simulink model "pro_newton1"  (R2022a)
settings: Solver=ode45  StartTime=0.0  StopTime=10.0  RelTol=1e-3
settings Model: Creator=55062  LastModifiedBy=55062
settings SolverCC: InitialStep=0.001

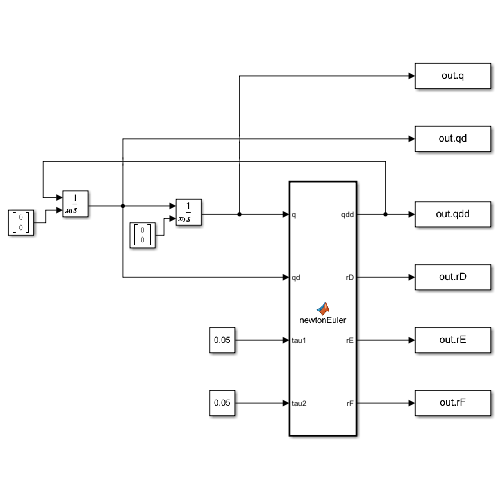
[thumbnail: Simulink's stored preview of the top-level diagram]
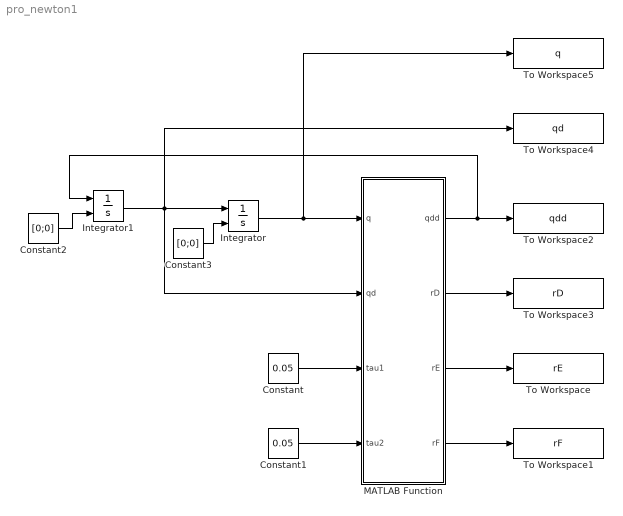
== system pro_newton1 ==
  Constant : Constant  Value=0.05
  Constant1 : Constant  Value=0.05
  Constant2 : Constant  Value=[0;0]  VectorParams1D=off
  Constant3 : Constant  Value=[0;0]  VectorParams1D=off
  Integrator : Integrator  InitialConditionSource=external
  Integrator1 : Integrator  InitialConditionSource=external
  MATLAB Function : MATLAB Function  TreatAsAtomicUnit=on
  To Workspace : ToWorkspace  VariableName=rE  SaveFormat=Timeseries  SampleTime=-1
  To Workspace1 : ToWorkspace  VariableName=rF  SaveFormat=Timeseries  SampleTime=-1
  To Workspace2 : ToWorkspace  VariableName=qdd  SaveFormat=Timeseries  SampleTime=-1
  To Workspace3 : ToWorkspace  VariableName=rD  SaveFormat=Timeseries  SampleTime=-1
  To Workspace4 : ToWorkspace  VariableName=qd  SaveFormat=Timeseries  SampleTime=-1
  To Workspace5 : ToWorkspace  VariableName=q  SaveFormat=Timeseries  SampleTime=-1
  wires:
  Integrator/1 -> To Workspace5/1, MATLAB Function/1(q)
  Integrator1/1 -> MATLAB Function/2(qd), To Workspace4/1, Integrator/1
  MATLAB Function/1(qdd) -> To Workspace2/1, Integrator1/1
  Constant/1 -> MATLAB Function/3(tau1)
  Constant1/1 -> MATLAB Function/4(tau2)
  MATLAB Function/3(rE) -> To Workspace/1
  MATLAB Function/4(rF) -> To Workspace1/1
  MATLAB Function/2(rD) -> To Workspace3/1
  Constant2/1 -> Integrator1/2
  Constant3/1 -> Integrator/2

== matlab function pro_newton1/MATLAB Function ==
  data: qdd output; rD output; q input; qd input; tau1 input; tau2 input; rE output; rF output
function [qdd,rD,rE,rF]  = newtonEuler(q,qd,tau1,tau2)
L0 = 0.5;
L1 = 0.15;
L2 = 0.1;
m1 = 0.6;
m2 = 0.5;
J1 = m1*L1^2/12;
J2 = m2*L2^2/12;
g = 9.8;
II = [0,-1;1,0];
ex = [1;0];

l1 = 0.05;
l2 = 0.025;

R1 = [cos(q(1)), -sin(q(1)); sin(q(1)), cos(q(1))];
R2 = [cos(q(2)), -sin(q(2)); sin(q(2)), cos(q(2))];
rC = [L0;0];
rD = rC - l1*R1*ex;
rE = rC + (L1 - l1)*R1*ex;
rF = rC - l1*R1*ex + L2*R2*ex/2;

J = [(L1/2-l1)*II*R1*ex, zeros(2,1);...
     1,                  0;...
     -l1*II*R1*ex,       (L2/2-l2)*II*R2*ex;...
     0,                  1];

C = [-(L1/2-l1)*R1*ex*(qd(1)^2);...
     0;...
     l1*R1*ex*(qd(1)^2) - (L2/2-l2)*R2*ex*(qd(2)^2);...
     0];

Phi = diag([m1,m1,J1,m2,m2,J2]);

F = [0;-m1*g;-tau1*qd(1);0;-m2*g;-tau2*qd(2)];

qdd = (J'*Phi*J)\(J'*(F - C));

end
